simulink model "SIL_OlfatiSaber"  (R2021b)
settings: Solver=FixedStepDiscrete  StartTime=0  StopTime=T  FixedStep=0.01  RelTol=1e-3  EnableMultiTasking=on
model workspace (MAT data in the model file):
  SL_ROS_VariableLengthArrays_MaxSizes : object (value not decoded)
values from neighbouring files (symbols this model uses):
  airspeed_ref = 42    [start_swarm.m]
  altitude_ref = 300    [start_swarm.m]
  N_Waypoints = size(Waypoints,1)    [start_swarm.m]
  radius_waypoint = 200    [start_swarm.m]
  Waypoints = [1200 -1000 ... (first row only)    [start_swarm.m]
undefined symbols (not defined in the file or in its folder): DiscIntNeverNeededParam, Elevators, p_swarm, Propeller, RightAileron, RightFlap, Rudder
libraries: robotlib x36, slpidlib x15, eeGeneralControl x5, simulink x5
(part 2 of 5)

== system SIL_OlfatiSaber/UAV 2/High-level/Waypoint Generator ==
  Xi : Inport
  Pos_i : Inport  Port=2
  Constant : Constant  Value=radius_waypoint
  Constant1 : Constant  Value=Waypoints
  Constant2 : Constant  Value=N_Waypoints
  Constant3 : Constant  Value=p_swarm.r
  Display : Display
  Memory : Memory
  Velocity Direction : MATLAB Function  TreatAsAtomicUnit=on
  Waypoint Algorithm : MATLAB Function  TreatAsAtomicUnit=on
  u : Outport
  wires:
  Memory/1 -> Waypoint Algorithm/6("Current_Waypoint ")
  Constant1/1 -> Waypoint Algorithm/4(Waypoints)
  Xi/1 -> Waypoint Algorithm/1(Xi)
  Constant3/1 -> Waypoint Algorithm/3(p_swarm_r)
  Constant2/1 -> Waypoint Algorithm/5(N_Waypoints)
  Waypoint Algorithm/2(Current_Waypoint) -> Memory/1, Display/1
  Constant/1 -> Waypoint Algorithm/2(R)
  Pos_i/1 -> Velocity Direction/1(pos)
  Velocity Direction/1(u_ref) -> u/1
  Waypoint Algorithm/1(wp) -> Velocity Direction/2(wp)

== system SIL_OlfatiSaber/UAV 2/Low-level/Autopilot ==
  note: bota po
  vel ref : Inport
  Euler angles : Inport  Port=2
  roll_ref : Inport  Port=3
  altitude : Inport  Port=4
  vel_in : Inport  Port=5
  altitude ref : Inport  Port=6
  Altitude Control : Subsystem
      settings: PortSchema="{\"entries\":[{\"content\":{\"sides\":[{\"content\":{\"connectorIds\":[\"In1\",\"In2\"]},\"type\":\"ConnectorPlacement.EquallySpacedRectSide\",\"uuid\":\"98c80c82-2588-492a-897d-d133440579b3\"},{\"content\":{\"connectorIds\":[\"Out1\"],\"side\":\"RIGHT\"},\"type\":\"ConnectorPlacement.EquallySpacedRectSide\",\"uuid\":\"157fcffb-564d-4941-a636-42e4165df758\"},{\"content\":{\"connectorIds\":[\"Out2\"],\"side\":\"TOP\"},\"type\":\"ConnectorPlacement.EquallySpacedRectSide\",\"uuid\":\"44b57248-226e-45fd-814c-d7eb072c2d1f\"},{\"content\":{\"connectorIds\":[],\"side\":\"HIDDEN\"},\"type\":\"ConnectorPlacement.EquallySpacedRectSide\",\"uuid\":\"dff6d6ab-ae11-4516-9107-00b7ae45fb5b\"}]},\"type\":\"ConnectorPlacement.EquallySpacedConnector\",\"uuid\":\"b6a62117-e3d4-4c2a-a3b5-b134a2ba950a\"}],\"packageUris\":[\"http://schema.mathworks.com/mf0/Connector/R2020b\"],\"version\":\"1.0\"}"
  Attitude Control : Subsystem
  Constant : Constant  Value=0
  Saturation2 : Saturate  UpperLimit=0.0523599  LowerLimit=-0.0523599
  Saturation3 : Saturate  UpperLimit=0.8  LowerLimit=0.6
  Saturation4 : Saturate  UpperLimit=0.0523599  LowerLimit=-0.0523599
  Takeoff : Subsystem  Commented=on
  Velocity Control : Subsystem
      settings: PortSchema="{\"entries\":[{\"content\":{\"sides\":[{\"content\":{\"connectorIds\":[\"In1\",\"In2\"]},\"type\":\"ConnectorPlacement.EquallySpacedRectSide\",\"uuid\":\"98c80c82-2588-492a-897d-d133440579b3\"},{\"content\":{\"connectorIds\":[\"Out1\"],\"side\":\"RIGHT\"},\"type\":\"ConnectorPlacement.EquallySpacedRectSide\",\"uuid\":\"157fcffb-564d-4941-a636-42e4165df758\"},{\"content\":{\"connectorIds\":[\"Out2\"],\"side\":\"TOP\"},\"type\":\"ConnectorPlacement.EquallySpacedRectSide\",\"uuid\":\"44b57248-226e-45fd-814c-d7eb072c2d1f\"},{\"content\":{\"connectorIds\":[],\"side\":\"HIDDEN\"},\"type\":\"ConnectorPlacement.EquallySpacedRectSide\",\"uuid\":\"dff6d6ab-ae11-4516-9107-00b7ae45fb5b\"}]},\"type\":\"ConnectorPlacement.EquallySpacedConnector\",\"uuid\":\"b6a62117-e3d4-4c2a-a3b5-b134a2ba950a\"}],\"packageUris\":[\"http://schema.mathworks.com/mf0/Connector/R2020b\"],\"version\":\"1.0\"}"
  profundor_cmd : Outport
  rudder_cmd : Outport  Port=2
  aileron_cmd : Outport  Port=3
  propeller_cmd : Outport  Port=4
  alt_e : Outport  Port=5
  vel_e : Outport  Port=6
  roll_e : Outport  Port=7
  pitch_e : Outport  Port=8
  wires:
  vel ref/1 -> Velocity Control/1(Velocity Ref)
  altitude ref/1 -> Altitude Control/1(Altitude Ref)
  vel_in/1 -> Velocity Control/2(Velocity)
  Altitude Control/2(altitude_error) -> alt_e/1
  Velocity Control/2(velocity_error) -> vel_e/1
  Altitude Control/1(Pitch_ref) -> Attitude Control/1(Pitch Ref)
  roll_ref/1 -> Attitude Control/2(Roll_ref)
  Euler angles/1 -> Attitude Control/3(Euler angles)
  Attitude Control/1(pitch_error) -> pitch_e/1, Saturation4/1
  Attitude Control/2(roll_error) -> Saturation2/1, roll_e/1
  Velocity Control/1(propeller_cmd) -> Saturation3/1
  Saturation3/1 -> propeller_cmd/1
  Saturation2/1 -> aileron_cmd/1
  Saturation4/1 -> profundor_cmd/1
  altitude/1 -> Altitude Control/2(Altitude)
  Constant/1 -> rudder_cmd/1

== system SIL_OlfatiSaber/UAV 2/Low-level/Guidance Algorithm ==
  yaw : Inport
  x : Inport  Port=2
  y : Inport  Port=3
  x ref : Inport  Port=4
  y ref : Inport  Port=5
  Atan2 : Trigonometry  Operator=atan2
  Constant : Constant
  Constant1 : Constant  Value=0
  Constant2 : Constant  Value=1.2
  Constant3 : Constant  Value=10
  Discrete PID : slpidlib/PID Controller  Controller=PID  Form=Parallel  TimeDomain=Discrete-time  UseExternalTs=off  SampleTime=-1  IntegratorMethod=Forward Euler  FilterMethod=Forward Euler  ControllerParametersSource=external  P=1  I=1  D=0  UseFilter=on  N=100  TunerSelectOption=Transfer Function Based (PID Tuner App)  InitialConditionSource=internal  InitialConditionForIntegrator=0  InitialConditionForFilter=0  DifferentiatorICPrevScaledInput=0  ExternalReset=none  TrackingMode=off  Kt=1  LimitOutput=off  SatLimitsSource=internal  UpperSaturationLimit=inf  LowerSaturationLimit=-inf  LinearizeAsGain=on  AntiWindupMode=none  Kb=1  POutMin=[]  POutMax=[]  IOutMin=[]  IOutMax=[]  DOutMin=[]  DOutMax=[]  NOutMin=[]  NOutMax=[]  SumOutMin=[]  SumOutMax=[]  SaturationOutMin=[]  SaturationOutMax=[]  PParamMin=[]  PParamMax=[]  IParamMin=[]  IParamMax=[]  DParamMin=[]  DParamMax=[]  NParamMin=[]  NParamMax=[]  KbParamMin=[]  KbParamMax=[]  KtParamMin=[]  KtParamMax=[]  KbOutMin=[]  KbOutMax=[]  KtOutMin=[]  KtOutMax=[]  IntegratorOutMin=[]  IntegratorOutMax=[]  FilterOutMin=[]  FilterOutMax=[]  SumI1OutMin=[]  SumI1OutMax=[]  SumI2OutMin=[]  SumI2OutMax=[]  SumI3OutMin=[]  SumI3OutMax=[]  SumI4OutMin=[]  SumI4OutMax=[]  SumDOutMin=[]  SumDOutMax=[]  DifferentiatorOutMin=[]  DifferentiatorOutMax=[]  FilterDiffOutCoefMin=[]  FilterDiffOutCoefMax=[]  ReciprocalOutMin=[]  ReciprocalOutMax=[]  SumDenOutMin=[]  SumDenOutMax=[]  SumNumOutMin=[]  SumNumOutMax=[]  DivideOutMin=[]  DivideOutMax=[]  UdiffTsProdOutMin=[]  UdiffTsProdOutMax=[]  NTsProdOutMin=[]  NTsProdOutMax=[]  UintegralTsProdOutMin=[]  UintegralTsProdOutMax=[]  UngainTsProdOutMin=[]  UngainTsProdOutMax=[]  IntegratorContinuousStateAttributes=''  IntegratorStateMustResolveToSignalObject=off  IntegratorRTWStateStorageClass=Auto  FilterContinuousStateAttributes=''  FilterStateMustResolveToSignalObject=off  FilterRTWStateStorageClass=Auto  ParallelPVariant=ExternalParameters  IdealPVariant=Disabled  IVariant=ExternalParameters  DVariant=ExternalParameters  IntegratorVariant=Discrete  SatVariant=Disabled  AWVariant=Passthrough  PCopyVariant=Disabled  TRVariant=Disabled  FdbkBlocksVariant=Forward  IdealPFdbkVariant=Disabled  SatFdbkVariant=Disabled  DerivativeFilterVariant=ForwardEulerFilter  NVariant=ExternalParameters  NCopyVariant=Disabled  FilterICVariant=InternalICsFilter  IntegratorICVariant=InternalICs  ExternalResetVariant=Disabled  TRSumVariant=Passthrough  SumFdbkVariant=Disabled  SumVariant=Sum_PID  TsampFilterVariant=InternalTs  TsampNgainVariant=Passthrough  TsampIntegralVariant=Passthrough  ExternalSaturationOutDataTypeStr=Inherit: Same as second input
  Gain : Gain  Gain=1.67
  Gain1 : Gain  Gain=-1
  Mux1 : Mux  Inputs=2
  Mux2 : Mux  Inputs=2
  Mux3 : Mux  Inputs=2
  Saturation : Saturate  UpperLimit=0.226893  LowerLimit=-0.226893
  Sum2 : Sum  Inputs=|+-
  Sum3 : Sum  Inputs=|+-
  Sum4 : Sum  Inputs=|+-
  roll_ref : Outport
  yaw_error : Outport  Port=2
  positions : Outport  Port=3
  wires:
  Mux1/1 -> Mux3/1
  Mux2/1 -> Mux3/2
  Saturation/1 -> Gain1/1
  Sum3/1 -> Atan2/1
  y/1 -> Sum3/2, Mux2/2
  y ref/1 -> Mux2/1, Sum3/1
  x ref/1 -> Mux1/1, Sum2/1
  x/1 -> Sum2/2, Mux1/2
  Sum2/1 -> Atan2/2
  Atan2/1 -> Sum4/1
  yaw/1 -> Sum4/2
  Mux3/1 -> positions/1
  Discrete PID/1 -> Saturation/1
  Sum4/1 -> yaw_error/1, Gain/1
  Gain1/1 -> roll_ref/1
  Constant/1 -> Discrete PID/2
  Constant1/1 -> Discrete PID/3
  Constant2/1 -> Discrete PID/4
  Constant3/1 -> Discrete PID/5
  Gain/1 -> Discrete PID/1

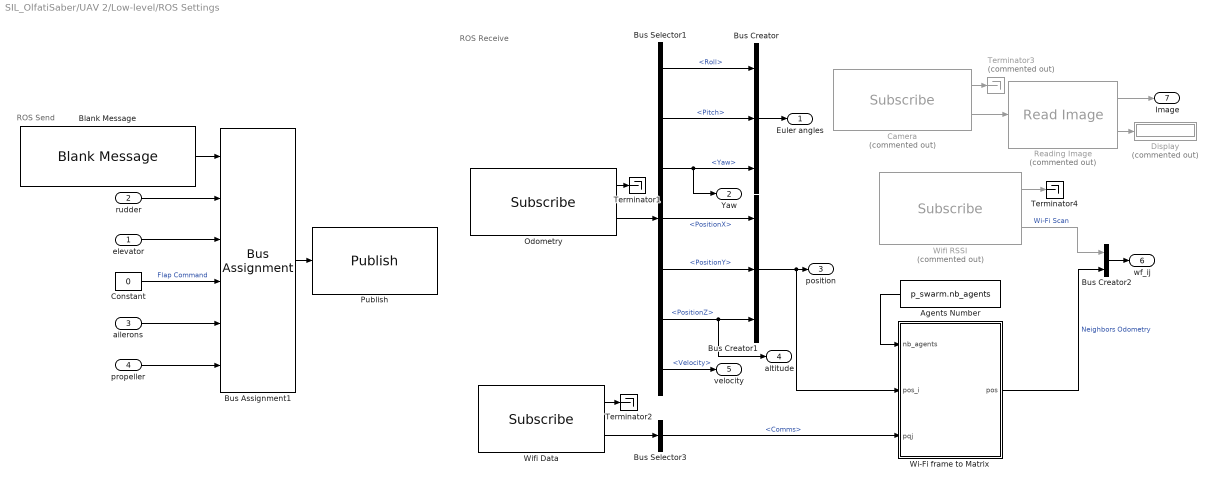
== system SIL_OlfatiSaber/UAV 2/Low-level/ROS Settings ==
  note: ROS Receive
  note: ROS Send
  elevator : Inport
  rudder : Inport  Port=2
  ailerons : Inport  Port=3
  propeller : Inport  Port=4
  Agents Number : Constant  Value=p_swarm.nb_agents
  Blank Message : robotlib/Blank Message  messageClass=Message  entityType=cosmus_messages/Control_Surfaces  messageType=cosmus_messages/Control_Surfaces  SampleTime=-1  legacyBusStruct=off
  Bus Assignment1 : BusAssignment  AssignedSignals=Rudder,Elevators,RightFlap,RightAileron,Propeller
  Bus Creator : BusCreator  Inputs=3
  Bus Creator1 : BusCreator  Inputs=3
  Bus Creator2 : BusCreator  Inputs=2
  Bus Selector1 : BusSelector  OutputSignals=Roll,Pitch,Yaw,PositionX,PositionY,PositionZ,Velocity
  Bus Selector3 : BusSelector  OutputSignals=Comms
  Camera : robotlib/Subscribe  Commented=on  topicSource=Select from ROS network  topic=/uav1/camera/image_raw  messageType=sensor_msgs/Image  SampleTime=-1  legacyBusStruct=off  messageQueueLength=1
  Constant : Constant  Value=0
  Display : Display  Commented=on
  Odometry : robotlib/Subscribe  topicSource=Select from ROS network  topic=/uav2/ground_truth/Odometry  messageType=cosmus_communication/Odom  SampleTime=-1  legacyBusStruct=off  messageQueueLength=1
  Publish : robotlib/Publish  topicSource=Select from ROS network  topic=/uav2/command  messageType=cosmus_messages/Control_Surfaces  legacyBusStruct=off  messageQueueLength=1
  Reading Image : robotlib/Read Image  Commented=on  MaximumImageSize=[240, 360]  ImageEncoding=rgb8  ShowAlphaOutput=off  ShowErrorCodeOutput=on  VariableSizeOutputs=off
      settings: SourceProductBaseCode=RR
  Terminator1 : Terminator
  Terminator2 : Terminator
  Terminator3 : Terminator  Commented=on
  Terminator4 : Terminator
  Wi-Fi frame to Matrix : MATLAB Function  TreatAsAtomicUnit=on
  Wifi Data : robotlib/Subscribe  topicSource=Select from ROS network  topic=/uav2/wifi_receiver/data  messageType=cosmus_messages/NetworkComm  SampleTime=-1  legacyBusStruct=off  messageQueueLength=1
  Wifi RSSI : robotlib/Subscribe  Commented=on  topicSource=Select from ROS network  topic=/uav1/wifi_receiver/wifi_scan  messageType=cosmus_messages/WifiSignals  SampleTime=-1  legacyBusStruct=off  messageQueueLength=1
  Euler angles : Outport
  Yaw : Outport  Port=2
  position : Outport  Port=3
  altitude : Outport  Port=4
  velocity : Outport  Port=5
  wf_ij : Outport  Port=6
  Image : Outport  Port=7
  wires:
  Odometry/1 -> Terminator1/1
  Blank Message/1 -> Bus Assignment1/1
  Bus Selector1/3 -> Bus Creator/3, Yaw/1  "<Yaw>"
  Bus Creator/1 -> Euler angles/1
  Bus Selector1/1 -> Bus Creator/1  "<Roll>"
  Bus Selector1/2 -> Bus Creator/2  "<Pitch>"
  Constant/1 -> Bus Assignment1/4  "Flap Command"
  Bus Assignment1/1 -> Publish/1
  Odometry/2 -> Bus Selector1/1
  Bus Selector1/4 -> Bus Creator1/1  "<PositionX>"
  Bus Selector1/5 -> Bus Creator1/2  "<PositionY>"
  Bus Selector1/6 -> Bus Creator1/3, altitude/1  "<PositionZ>"
  propeller/1 -> Bus Assignment1/6
  ailerons/1 -> Bus Assignment1/5
  elevator/1 -> Bus Assignment1/3
  Bus Selector1/7 -> velocity/1  "<Velocity>"
  rudder/1 -> Bus Assignment1/2
  Wifi Data/1 -> Terminator2/1
  Wifi Data/2 -> Bus Selector3/1
  Bus Selector3/1 -> Wi-Fi frame to Matrix/3(pqj)  "<Comms>"
  Agents Number/1 -> Wi-Fi frame to Matrix/1(nb_agents)
  Bus Creator1/1 -> position/1, Wi-Fi frame to Matrix/2(pos_i)
  Wi-Fi frame to Matrix/1(pos) -> Bus Creator2/2  "Neighbors Odometry"
  Camera/2 -> Reading Image/1
  Reading Image/1 -> Image/1
  Reading Image/2 -> Display/1
  Camera/1 -> Terminator3/1
  Wifi RSSI/1 -> Terminator4/1
  Wifi RSSI/2 -> Bus Creator2/1  "Wi-Fi Scan"
  Bus Creator2/1 -> wf_ij/1

== system SIL_OlfatiSaber/UAV 2/Low-level/Vision ==
  Image : Inport
  Video Viewer : VideoViewer  Commented=on  FigPos=[505 744 418 304]
  wires:
  Image/1 -> Video Viewer/1

== system SIL_OlfatiSaber/UAV 3/High-level/Coordination Algorithm ==
  Xi : Inport
  u : Inport  Port=2
  Demux : Demux  Outputs=3
  Discrete Derivative : simulink/Discrete/Discrete Derivative  gainval=1.0  ICPrevScaledInput=0.0  OutMin=[]  OutMax=[]  OutDataType=fixdt(1, 16)  OutScaling=2^-10  DoSatur=off
  Discrete-Time Integrator : DiscreteIntegrator  SampleTime=-1  ICPrevOutput=DiscIntNeverNeededParam  ICPrevScaledInput=DiscIntNeverNeededParam
  Olfati-Saber Algorithm : MATLAB Function  TreatAsAtomicUnit=on
  Parameters : Subsystem
  dt : Constant  Value=0.01
  r_agent : Constant  Value=p_swarm.r_agent
  X : Outport
  Y : Outport  Port=2
  Z : Outport  Port=3
  wires:
  Olfati-Saber Algorithm/1(vel_command) -> Discrete-Time Integrator/1
  dt/1 -> Olfati-Saber Algorithm/5(dt)
  r_agent/1 -> Olfati-Saber Algorithm/6(r_agent)
  Discrete-Time Integrator/1 -> Demux/1
  Demux/2 -> Y/1
  Demux/1 -> X/1
  Demux/3 -> Z/1
  Discrete Derivative/1 -> Olfati-Saber Algorithm/3(vel)
  Parameters/1(p_swarm) -> Olfati-Saber Algorithm/1(p_swarm_par)
  Xi/1 -> Discrete Derivative/1, Olfati-Saber Algorithm/2(pos)
  u/1 -> Olfati-Saber Algorithm/4(u_ref)

== system SIL_OlfatiSaber/UAV 3/High-level/Network ==
  Scan : Inport
  Agents Number : Constant  Value=p_swarm.nb_agents
  Bus Selector : BusSelector  OutputSignals=Neighbors Odometry,Wi-Fi Scan
  Status Network : MATLAB Function  Commented=on  TreatAsAtomicUnit=on
  Terminator5 : Terminator
  Pos_J : Outport
  wires:
  Status Network/1(SignalDbms) -> Terminator5/1
  Agents Number/1 -> Status Network/1(N_Agents)
  Scan/1 -> Bus Selector/1
  Bus Selector/1 -> Pos_J/1  "<Neighbors Odometry>"
  Bus Selector/2 -> Status Network/2(Wifi_Scan)  "<Wi-Fi Scan>"

== system SIL_OlfatiSaber/UAV 3/High-level/Waypoint Generator ==
  Xi : Inport
  Pos_i : Inport  Port=2
  Constant : Constant  Value=radius_waypoint
  Constant1 : Constant  Value=Waypoints
  Constant2 : Constant  Value=N_Waypoints
  Constant3 : Constant  Value=p_swarm.r
  Display : Display
  Memory : Memory
  Velocity Direction : MATLAB Function  TreatAsAtomicUnit=on
  Waypoint Algorithm : MATLAB Function  TreatAsAtomicUnit=on
  u : Outport
  wires:
  Memory/1 -> Waypoint Algorithm/6("Current_Waypoint ")
  Constant1/1 -> Waypoint Algorithm/4(Waypoints)
  Xi/1 -> Waypoint Algorithm/1(Xi)
  Constant3/1 -> Waypoint Algorithm/3(p_swarm_r)
  Constant2/1 -> Waypoint Algorithm/5(N_Waypoints)
  Waypoint Algorithm/2(Current_Waypoint) -> Memory/1, Display/1
  Constant/1 -> Waypoint Algorithm/2(R)
  Pos_i/1 -> Velocity Direction/1(pos)
  Velocity Direction/1(u_ref) -> u/1
  Waypoint Algorithm/1(wp) -> Velocity Direction/2(wp)

== system SIL_OlfatiSaber/UAV 3/Low-level/Autopilot ==
  note: bota po
  vel ref : Inport
  Euler angles : Inport  Port=2
  roll_ref : Inport  Port=3
  altitude : Inport  Port=4
  vel_in : Inport  Port=5
  altitude ref : Inport  Port=6
  Altitude Control : Subsystem
      settings: PortSchema="{\"entries\":[{\"content\":{\"sides\":[{\"content\":{\"connectorIds\":[\"In1\",\"In2\"]},\"type\":\"ConnectorPlacement.EquallySpacedRectSide\",\"uuid\":\"98c80c82-2588-492a-897d-d133440579b3\"},{\"content\":{\"connectorIds\":[\"Out1\"],\"side\":\"RIGHT\"},\"type\":\"ConnectorPlacement.EquallySpacedRectSide\",\"uuid\":\"157fcffb-564d-4941-a636-42e4165df758\"},{\"content\":{\"connectorIds\":[\"Out2\"],\"side\":\"TOP\"},\"type\":\"ConnectorPlacement.EquallySpacedRectSide\",\"uuid\":\"44b57248-226e-45fd-814c-d7eb072c2d1f\"},{\"content\":{\"connectorIds\":[],\"side\":\"HIDDEN\"},\"type\":\"ConnectorPlacement.EquallySpacedRectSide\",\"uuid\":\"dff6d6ab-ae11-4516-9107-00b7ae45fb5b\"}]},\"type\":\"ConnectorPlacement.EquallySpacedConnector\",\"uuid\":\"b6a62117-e3d4-4c2a-a3b5-b134a2ba950a\"}],\"packageUris\":[\"http://schema.mathworks.com/mf0/Connector/R2020b\"],\"version\":\"1.0\"}"
  Attitude Control : Subsystem
  Constant : Constant  Value=0
  Saturation2 : Saturate  UpperLimit=0.0523599  LowerLimit=-0.0523599
  Saturation3 : Saturate  UpperLimit=0.8  LowerLimit=0.6
  Saturation4 : Saturate  UpperLimit=0.0523599  LowerLimit=-0.0523599
  Takeoff : Subsystem  Commented=on
  Velocity Control : Subsystem
      settings: PortSchema="{\"entries\":[{\"content\":{\"sides\":[{\"content\":{\"connectorIds\":[\"In1\",\"In2\"]},\"type\":\"ConnectorPlacement.EquallySpacedRectSide\",\"uuid\":\"98c80c82-2588-492a-897d-d133440579b3\"},{\"content\":{\"connectorIds\":[\"Out1\"],\"side\":\"RIGHT\"},\"type\":\"ConnectorPlacement.EquallySpacedRectSide\",\"uuid\":\"157fcffb-564d-4941-a636-42e4165df758\"},{\"content\":{\"connectorIds\":[\"Out2\"],\"side\":\"TOP\"},\"type\":\"ConnectorPlacement.EquallySpacedRectSide\",\"uuid\":\"44b57248-226e-45fd-814c-d7eb072c2d1f\"},{\"content\":{\"connectorIds\":[],\"side\":\"HIDDEN\"},\"type\":\"ConnectorPlacement.EquallySpacedRectSide\",\"uuid\":\"dff6d6ab-ae11-4516-9107-00b7ae45fb5b\"}]},\"type\":\"ConnectorPlacement.EquallySpacedConnector\",\"uuid\":\"b6a62117-e3d4-4c2a-a3b5-b134a2ba950a\"}],\"packageUris\":[\"http://schema.mathworks.com/mf0/Connector/R2020b\"],\"version\":\"1.0\"}"
  profundor_cmd : Outport
  rudder_cmd : Outport  Port=2
  aileron_cmd : Outport  Port=3
  propeller_cmd : Outport  Port=4
  alt_e : Outport  Port=5
  vel_e : Outport  Port=6
  roll_e : Outport  Port=7
  pitch_e : Outport  Port=8
  wires:
  vel ref/1 -> Velocity Control/1(Velocity Ref)
  altitude ref/1 -> Altitude Control/1(Altitude Ref)
  vel_in/1 -> Velocity Control/2(Velocity)
  Altitude Control/2(altitude_error) -> alt_e/1
  Velocity Control/2(velocity_error) -> vel_e/1
  Altitude Control/1(Pitch_ref) -> Attitude Control/1(Pitch Ref)
  roll_ref/1 -> Attitude Control/2(Roll_ref)
  Euler angles/1 -> Attitude Control/3(Euler angles)
  Attitude Control/1(pitch_error) -> pitch_e/1, Saturation4/1
  Attitude Control/2(roll_error) -> Saturation2/1, roll_e/1
  Velocity Control/1(propeller_cmd) -> Saturation3/1
  Saturation3/1 -> propeller_cmd/1
  Saturation2/1 -> aileron_cmd/1
  Saturation4/1 -> profundor_cmd/1
  altitude/1 -> Altitude Control/2(Altitude)
  Constant/1 -> rudder_cmd/1

== system SIL_OlfatiSaber/UAV 3/Low-level/Guidance Algorithm ==
  yaw : Inport
  x : Inport  Port=2
  y : Inport  Port=3
  x ref : Inport  Port=4
  y ref : Inport  Port=5
  Atan2 : Trigonometry  Operator=atan2
  Constant : Constant
  Constant1 : Constant  Value=0
  Constant2 : Constant  Value=1.2
  Constant3 : Constant  Value=10
  Discrete PID : slpidlib/PID Controller  Controller=PID  Form=Parallel  TimeDomain=Discrete-time  UseExternalTs=off  SampleTime=-1  IntegratorMethod=Forward Euler  FilterMethod=Forward Euler  ControllerParametersSource=external  P=1  I=1  D=0  UseFilter=on  N=100  TunerSelectOption=Transfer Function Based (PID Tuner App)  InitialConditionSource=internal  InitialConditionForIntegrator=0  InitialConditionForFilter=0  DifferentiatorICPrevScaledInput=0  ExternalReset=none  TrackingMode=off  Kt=1  LimitOutput=off  SatLimitsSource=internal  UpperSaturationLimit=inf  LowerSaturationLimit=-inf  LinearizeAsGain=on  AntiWindupMode=none  Kb=1  POutMin=[]  POutMax=[]  IOutMin=[]  IOutMax=[]  DOutMin=[]  DOutMax=[]  NOutMin=[]  NOutMax=[]  SumOutMin=[]  SumOutMax=[]  SaturationOutMin=[]  SaturationOutMax=[]  PParamMin=[]  PParamMax=[]  IParamMin=[]  IParamMax=[]  DParamMin=[]  DParamMax=[]  NParamMin=[]  NParamMax=[]  KbParamMin=[]  KbParamMax=[]  KtParamMin=[]  KtParamMax=[]  KbOutMin=[]  KbOutMax=[]  KtOutMin=[]  KtOutMax=[]  IntegratorOutMin=[]  IntegratorOutMax=[]  FilterOutMin=[]  FilterOutMax=[]  SumI1OutMin=[]  SumI1OutMax=[]  SumI2OutMin=[]  SumI2OutMax=[]  SumI3OutMin=[]  SumI3OutMax=[]  SumI4OutMin=[]  SumI4OutMax=[]  SumDOutMin=[]  SumDOutMax=[]  DifferentiatorOutMin=[]  DifferentiatorOutMax=[]  FilterDiffOutCoefMin=[]  FilterDiffOutCoefMax=[]  ReciprocalOutMin=[]  ReciprocalOutMax=[]  SumDenOutMin=[]  SumDenOutMax=[]  SumNumOutMin=[]  SumNumOutMax=[]  DivideOutMin=[]  DivideOutMax=[]  UdiffTsProdOutMin=[]  UdiffTsProdOutMax=[]  NTsProdOutMin=[]  NTsProdOutMax=[]  UintegralTsProdOutMin=[]  UintegralTsProdOutMax=[]  UngainTsProdOutMin=[]  UngainTsProdOutMax=[]  IntegratorContinuousStateAttributes=''  IntegratorStateMustResolveToSignalObject=off  IntegratorRTWStateStorageClass=Auto  FilterContinuousStateAttributes=''  FilterStateMustResolveToSignalObject=off  FilterRTWStateStorageClass=Auto  ParallelPVariant=ExternalParameters  IdealPVariant=Disabled  IVariant=ExternalParameters  DVariant=ExternalParameters  IntegratorVariant=Discrete  SatVariant=Disabled  AWVariant=Passthrough  PCopyVariant=Disabled  TRVariant=Disabled  FdbkBlocksVariant=Forward  IdealPFdbkVariant=Disabled  SatFdbkVariant=Disabled  DerivativeFilterVariant=ForwardEulerFilter  NVariant=ExternalParameters  NCopyVariant=Disabled  FilterICVariant=InternalICsFilter  IntegratorICVariant=InternalICs  ExternalResetVariant=Disabled  TRSumVariant=Passthrough  SumFdbkVariant=Disabled  SumVariant=Sum_PID  TsampFilterVariant=InternalTs  TsampNgainVariant=Passthrough  TsampIntegralVariant=Passthrough  ExternalSaturationOutDataTypeStr=Inherit: Same as second input
  Gain : Gain  Gain=1.67
  Gain1 : Gain  Gain=-1
  Mux1 : Mux  Inputs=2
  Mux2 : Mux  Inputs=2
  Mux3 : Mux  Inputs=2
  Saturation : Saturate  UpperLimit=0.226893  LowerLimit=-0.226893
  Sum2 : Sum  Inputs=|+-
  Sum3 : Sum  Inputs=|+-
  Sum4 : Sum  Inputs=|+-
  roll_ref : Outport
  yaw_error : Outport  Port=2
  positions : Outport  Port=3
  wires:
  Mux1/1 -> Mux3/1
  Mux2/1 -> Mux3/2
  Saturation/1 -> Gain1/1
  Sum3/1 -> Atan2/1
  y/1 -> Sum3/2, Mux2/2
  y ref/1 -> Mux2/1, Sum3/1
  x ref/1 -> Mux1/1, Sum2/1
  x/1 -> Sum2/2, Mux1/2
  Sum2/1 -> Atan2/2
  Atan2/1 -> Sum4/1
  yaw/1 -> Sum4/2
  Mux3/1 -> positions/1
  Discrete PID/1 -> Saturation/1
  Sum4/1 -> yaw_error/1, Gain/1
  Gain1/1 -> roll_ref/1
  Constant/1 -> Discrete PID/2
  Constant1/1 -> Discrete PID/3
  Constant2/1 -> Discrete PID/4
  Constant3/1 -> Discrete PID/5
  Gain/1 -> Discrete PID/1

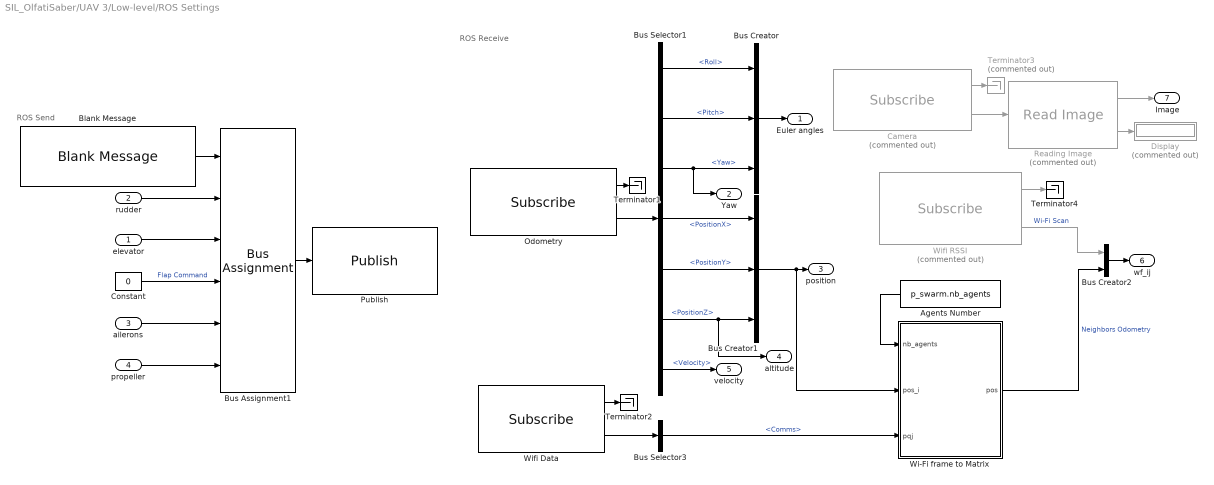
== system SIL_OlfatiSaber/UAV 3/Low-level/ROS Settings ==
  note: ROS Receive
  note: ROS Send
  elevator : Inport
  rudder : Inport  Port=2
  ailerons : Inport  Port=3
  propeller : Inport  Port=4
  Agents Number : Constant  Value=p_swarm.nb_agents
  Blank Message : robotlib/Blank Message  messageClass=Message  entityType=cosmus_messages/Control_Surfaces  messageType=cosmus_messages/Control_Surfaces  SampleTime=-1  legacyBusStruct=off
  Bus Assignment1 : BusAssignment  AssignedSignals=Rudder,Elevators,RightFlap,RightAileron,Propeller
  Bus Creator : BusCreator  Inputs=3
  Bus Creator1 : BusCreator  Inputs=3
  Bus Creator2 : BusCreator  Inputs=2
  Bus Selector1 : BusSelector  OutputSignals=Roll,Pitch,Yaw,PositionX,PositionY,PositionZ,Velocity
  Bus Selector3 : BusSelector  OutputSignals=Comms
  Camera : robotlib/Subscribe  Commented=on  topicSource=Select from ROS network  topic=/uav1/camera/image_raw  messageType=sensor_msgs/Image  SampleTime=-1  legacyBusStruct=off  messageQueueLength=1
  Constant : Constant  Value=0
  Display : Display  Commented=on
  Odometry : robotlib/Subscribe  topicSource=Select from ROS network  topic=/uav3/ground_truth/Odometry  messageType=cosmus_communication/Odom  SampleTime=-1  legacyBusStruct=off  messageQueueLength=1
  Publish : robotlib/Publish  topicSource=Select from ROS network  topic=/uav3/command  messageType=cosmus_messages/Control_Surfaces  legacyBusStruct=off  messageQueueLength=1
  Reading Image : robotlib/Read Image  Commented=on  MaximumImageSize=[240, 360]  ImageEncoding=rgb8  ShowAlphaOutput=off  ShowErrorCodeOutput=on  VariableSizeOutputs=off
      settings: SourceProductBaseCode=RR
  Terminator1 : Terminator
  Terminator2 : Terminator
  Terminator3 : Terminator  Commented=on
  Terminator4 : Terminator
  Wi-Fi frame to Matrix : MATLAB Function  TreatAsAtomicUnit=on
  Wifi Data : robotlib/Subscribe  topicSource=Select from ROS network  topic=/uav3/wifi_receiver/data  messageType=cosmus_messages/NetworkComm  SampleTime=-1  legacyBusStruct=off  messageQueueLength=1
  Wifi RSSI : robotlib/Subscribe  Commented=on  topicSource=Select from ROS network  topic=/uav1/wifi_receiver/wifi_scan  messageType=cosmus_messages/WifiSignals  SampleTime=-1  legacyBusStruct=off  messageQueueLength=1
  Euler angles : Outport
  Yaw : Outport  Port=2
  position : Outport  Port=3
  altitude : Outport  Port=4
  velocity : Outport  Port=5
  wf_ij : Outport  Port=6
  Image : Outport  Port=7
  wires:
  Odometry/1 -> Terminator1/1
  Blank Message/1 -> Bus Assignment1/1
  Bus Selector1/3 -> Bus Creator/3, Yaw/1  "<Yaw>"
  Bus Creator/1 -> Euler angles/1
  Bus Selector1/1 -> Bus Creator/1  "<Roll>"
  Bus Selector1/2 -> Bus Creator/2  "<Pitch>"
  Constant/1 -> Bus Assignment1/4  "Flap Command"
  Bus Assignment1/1 -> Publish/1
  Odometry/2 -> Bus Selector1/1
  Bus Selector1/4 -> Bus Creator1/1  "<PositionX>"
  Bus Selector1/5 -> Bus Creator1/2  "<PositionY>"
  Bus Selector1/6 -> Bus Creator1/3, altitude/1  "<PositionZ>"
  propeller/1 -> Bus Assignment1/6
  ailerons/1 -> Bus Assignment1/5
  elevator/1 -> Bus Assignment1/3
  Bus Selector1/7 -> velocity/1  "<Velocity>"
  rudder/1 -> Bus Assignment1/2
  Wifi Data/1 -> Terminator2/1
  Wifi Data/2 -> Bus Selector3/1
  Bus Selector3/1 -> Wi-Fi frame to Matrix/3(pqj)  "<Comms>"
  Agents Number/1 -> Wi-Fi frame to Matrix/1(nb_agents)
  Bus Creator1/1 -> position/1, Wi-Fi frame to Matrix/2(pos_i)
  Wi-Fi frame to Matrix/1(pos) -> Bus Creator2/2  "Neighbors Odometry"
  Camera/2 -> Reading Image/1
  Reading Image/1 -> Image/1
  Reading Image/2 -> Display/1
  Camera/1 -> Terminator3/1
  Wifi RSSI/1 -> Terminator4/1
  Wifi RSSI/2 -> Bus Creator2/1  "Wi-Fi Scan"
  Bus Creator2/1 -> wf_ij/1

== system SIL_OlfatiSaber/UAV 3/Low-level/Vision ==
  Image : Inport
  Video Viewer : VideoViewer  Commented=on  FigPos=[505 744 418 304]
  wires:
  Image/1 -> Video Viewer/1

== system SIL_OlfatiSaber/UAV 4/High-level/Coordination Algorithm ==
  Xi : Inport
  u : Inport  Port=2
  Demux : Demux  Outputs=3
  Discrete Derivative : simulink/Discrete/Discrete Derivative  gainval=1.0  ICPrevScaledInput=0.0  OutMin=[]  OutMax=[]  OutDataType=fixdt(1, 16)  OutScaling=2^-10  DoSatur=off
  Discrete-Time Integrator : DiscreteIntegrator  SampleTime=-1  ICPrevOutput=DiscIntNeverNeededParam  ICPrevScaledInput=DiscIntNeverNeededParam
  Olfati-Saber Algorithm : MATLAB Function  TreatAsAtomicUnit=on
  Parameters : Subsystem
  dt : Constant  Value=0.01
  r_agent : Constant  Value=p_swarm.r_agent
  X : Outport
  Y : Outport  Port=2
  Z : Outport  Port=3
  wires:
  Olfati-Saber Algorithm/1(vel_command) -> Discrete-Time Integrator/1
  dt/1 -> Olfati-Saber Algorithm/5(dt)
  r_agent/1 -> Olfati-Saber Algorithm/6(r_agent)
  Discrete-Time Integrator/1 -> Demux/1
  Demux/2 -> Y/1
  Demux/1 -> X/1
  Demux/3 -> Z/1
  Discrete Derivative/1 -> Olfati-Saber Algorithm/3(vel)
  Parameters/1(p_swarm) -> Olfati-Saber Algorithm/1(p_swarm_par)
  Xi/1 -> Discrete Derivative/1, Olfati-Saber Algorithm/2(pos)
  u/1 -> Olfati-Saber Algorithm/4(u_ref)

== system SIL_OlfatiSaber/UAV 4/High-level/Network ==
  Scan : Inport
  Agents Number : Constant  Value=p_swarm.nb_agents
  Bus Selector : BusSelector  OutputSignals=Neighbors Odometry,Wi-Fi Scan
  Status Network : MATLAB Function  Commented=on  TreatAsAtomicUnit=on
  Terminator5 : Terminator
  Pos_J : Outport
  wires:
  Status Network/1(SignalDbms) -> Terminator5/1
  Agents Number/1 -> Status Network/1(N_Agents)
  Scan/1 -> Bus Selector/1
  Bus Selector/1 -> Pos_J/1  "<Neighbors Odometry>"
  Bus Selector/2 -> Status Network/2(Wifi_Scan)  "<Wi-Fi Scan>"

== system SIL_OlfatiSaber/UAV 4/High-level/Waypoint Generator ==
  Xi : Inport
  Pos_i : Inport  Port=2
  Constant : Constant  Value=radius_waypoint
  Constant1 : Constant  Value=Waypoints
  Constant2 : Constant  Value=N_Waypoints
  Constant3 : Constant  Value=p_swarm.r
  Display : Display
  Memory : Memory
  Velocity Direction : MATLAB Function  TreatAsAtomicUnit=on
  Waypoint Algorithm : MATLAB Function  TreatAsAtomicUnit=on
  u : Outport
  wires:
  Memory/1 -> Waypoint Algorithm/6("Current_Waypoint ")
  Constant1/1 -> Waypoint Algorithm/4(Waypoints)
  Xi/1 -> Waypoint Algorithm/1(Xi)
  Constant3/1 -> Waypoint Algorithm/3(p_swarm_r)
  Constant2/1 -> Waypoint Algorithm/5(N_Waypoints)
  Waypoint Algorithm/2(Current_Waypoint) -> Memory/1, Display/1
  Constant/1 -> Waypoint Algorithm/2(R)
  Pos_i/1 -> Velocity Direction/1(pos)
  Velocity Direction/1(u_ref) -> u/1
  Waypoint Algorithm/1(wp) -> Velocity Direction/2(wp)

== system SIL_OlfatiSaber/UAV 4/Low-level/Autopilot ==
  note: bota po
  vel ref : Inport
  Euler angles : Inport  Port=2
  roll_ref : Inport  Port=3
  altitude : Inport  Port=4
  vel_in : Inport  Port=5
  altitude ref : Inport  Port=6
  Altitude Control : Subsystem
      settings: PortSchema="{\"entries\":[{\"content\":{\"sides\":[{\"content\":{\"connectorIds\":[\"In1\",\"In2\"]},\"type\":\"ConnectorPlacement.EquallySpacedRectSide\",\"uuid\":\"98c80c82-2588-492a-897d-d133440579b3\"},{\"content\":{\"connectorIds\":[\"Out1\"],\"side\":\"RIGHT\"},\"type\":\"ConnectorPlacement.EquallySpacedRectSide\",\"uuid\":\"157fcffb-564d-4941-a636-42e4165df758\"},{\"content\":{\"connectorIds\":[\"Out2\"],\"side\":\"TOP\"},\"type\":\"ConnectorPlacement.EquallySpacedRectSide\",\"uuid\":\"44b57248-226e-45fd-814c-d7eb072c2d1f\"},{\"content\":{\"connectorIds\":[],\"side\":\"HIDDEN\"},\"type\":\"ConnectorPlacement.EquallySpacedRectSide\",\"uuid\":\"dff6d6ab-ae11-4516-9107-00b7ae45fb5b\"}]},\"type\":\"ConnectorPlacement.EquallySpacedConnector\",\"uuid\":\"b6a62117-e3d4-4c2a-a3b5-b134a2ba950a\"}],\"packageUris\":[\"http://schema.mathworks.com/mf0/Connector/R2020b\"],\"version\":\"1.0\"}"
  Attitude Control : Subsystem
  Constant : Constant  Value=0
  Saturation2 : Saturate  UpperLimit=0.0523599  LowerLimit=-0.0523599
  Saturation3 : Saturate  UpperLimit=0.8  LowerLimit=0.6
  Saturation4 : Saturate  UpperLimit=0.0523599  LowerLimit=-0.0523599
  Takeoff : Subsystem  Commented=on
  Velocity Control : Subsystem
      settings: PortSchema="{\"entries\":[{\"content\":{\"sides\":[{\"content\":{\"connectorIds\":[\"In1\",\"In2\"]},\"type\":\"ConnectorPlacement.EquallySpacedRectSide\",\"uuid\":\"98c80c82-2588-492a-897d-d133440579b3\"},{\"content\":{\"connectorIds\":[\"Out1\"],\"side\":\"RIGHT\"},\"type\":\"ConnectorPlacement.EquallySpacedRectSide\",\"uuid\":\"157fcffb-564d-4941-a636-42e4165df758\"},{\"content\":{\"connectorIds\":[\"Out2\"],\"side\":\"TOP\"},\"type\":\"ConnectorPlacement.EquallySpacedRectSide\",\"uuid\":\"44b57248-226e-45fd-814c-d7eb072c2d1f\"},{\"content\":{\"connectorIds\":[],\"side\":\"HIDDEN\"},\"type\":\"ConnectorPlacement.EquallySpacedRectSide\",\"uuid\":\"dff6d6ab-ae11-4516-9107-00b7ae45fb5b\"}]},\"type\":\"ConnectorPlacement.EquallySpacedConnector\",\"uuid\":\"b6a62117-e3d4-4c2a-a3b5-b134a2ba950a\"}],\"packageUris\":[\"http://schema.mathworks.com/mf0/Connector/R2020b\"],\"version\":\"1.0\"}"
  profundor_cmd : Outport
  rudder_cmd : Outport  Port=2
  aileron_cmd : Outport  Port=3
  propeller_cmd : Outport  Port=4
  alt_e : Outport  Port=5
  vel_e : Outport  Port=6
  roll_e : Outport  Port=7
  pitch_e : Outport  Port=8
  wires:
  vel ref/1 -> Velocity Control/1(Velocity Ref)
  altitude ref/1 -> Altitude Control/1(Altitude Ref)
  vel_in/1 -> Velocity Control/2(Velocity)
  Altitude Control/2(altitude_error) -> alt_e/1
  Velocity Control/2(velocity_error) -> vel_e/1
  Altitude Control/1(Pitch_ref) -> Attitude Control/1(Pitch Ref)
  roll_ref/1 -> Attitude Control/2(Roll_ref)
  Euler angles/1 -> Attitude Control/3(Euler angles)
  Attitude Control/1(pitch_error) -> pitch_e/1, Saturation4/1
  Attitude Control/2(roll_error) -> Saturation2/1, roll_e/1
  Velocity Control/1(propeller_cmd) -> Saturation3/1
  Saturation3/1 -> propeller_cmd/1
  Saturation2/1 -> aileron_cmd/1
  Saturation4/1 -> profundor_cmd/1
  altitude/1 -> Altitude Control/2(Altitude)
  Constant/1 -> rudder_cmd/1

== system SIL_OlfatiSaber/UAV 4/Low-level/Guidance Algorithm ==
  yaw : Inport
  x : Inport  Port=2
  y : Inport  Port=3
  x ref : Inport  Port=4
  y ref : Inport  Port=5
  Atan2 : Trigonometry  Operator=atan2
  Constant : Constant
  Constant1 : Constant  Value=0
  Constant2 : Constant  Value=1.2
  Constant3 : Constant  Value=10
  Discrete PID : slpidlib/PID Controller  Controller=PID  Form=Parallel  TimeDomain=Discrete-time  UseExternalTs=off  SampleTime=-1  IntegratorMethod=Forward Euler  FilterMethod=Forward Euler  ControllerParametersSource=external  P=1  I=1  D=0  UseFilter=on  N=100  TunerSelectOption=Transfer Function Based (PID Tuner App)  InitialConditionSource=internal  InitialConditionForIntegrator=0  InitialConditionForFilter=0  DifferentiatorICPrevScaledInput=0  ExternalReset=none  TrackingMode=off  Kt=1  LimitOutput=off  SatLimitsSource=internal  UpperSaturationLimit=inf  LowerSaturationLimit=-inf  LinearizeAsGain=on  AntiWindupMode=none  Kb=1  POutMin=[]  POutMax=[]  IOutMin=[]  IOutMax=[]  DOutMin=[]  DOutMax=[]  NOutMin=[]  NOutMax=[]  SumOutMin=[]  SumOutMax=[]  SaturationOutMin=[]  SaturationOutMax=[]  PParamMin=[]  PParamMax=[]  IParamMin=[]  IParamMax=[]  DParamMin=[]  DParamMax=[]  NParamMin=[]  NParamMax=[]  KbParamMin=[]  KbParamMax=[]  KtParamMin=[]  KtParamMax=[]  KbOutMin=[]  KbOutMax=[]  KtOutMin=[]  KtOutMax=[]  IntegratorOutMin=[]  IntegratorOutMax=[]  FilterOutMin=[]  FilterOutMax=[]  SumI1OutMin=[]  SumI1OutMax=[]  SumI2OutMin=[]  SumI2OutMax=[]  SumI3OutMin=[]  SumI3OutMax=[]  SumI4OutMin=[]  SumI4OutMax=[]  SumDOutMin=[]  SumDOutMax=[]  DifferentiatorOutMin=[]  DifferentiatorOutMax=[]  FilterDiffOutCoefMin=[]  FilterDiffOutCoefMax=[]  ReciprocalOutMin=[]  ReciprocalOutMax=[]  SumDenOutMin=[]  SumDenOutMax=[]  SumNumOutMin=[]  SumNumOutMax=[]  DivideOutMin=[]  DivideOutMax=[]  UdiffTsProdOutMin=[]  UdiffTsProdOutMax=[]  NTsProdOutMin=[]  NTsProdOutMax=[]  UintegralTsProdOutMin=[]  UintegralTsProdOutMax=[]  UngainTsProdOutMin=[]  UngainTsProdOutMax=[]  IntegratorContinuousStateAttributes=''  IntegratorStateMustResolveToSignalObject=off  IntegratorRTWStateStorageClass=Auto  FilterContinuousStateAttributes=''  FilterStateMustResolveToSignalObject=off  FilterRTWStateStorageClass=Auto  ParallelPVariant=ExternalParameters  IdealPVariant=Disabled  IVariant=ExternalParameters  DVariant=ExternalParameters  IntegratorVariant=Discrete  SatVariant=Disabled  AWVariant=Passthrough  PCopyVariant=Disabled  TRVariant=Disabled  FdbkBlocksVariant=Forward  IdealPFdbkVariant=Disabled  SatFdbkVariant=Disabled  DerivativeFilterVariant=ForwardEulerFilter  NVariant=ExternalParameters  NCopyVariant=Disabled  FilterICVariant=InternalICsFilter  IntegratorICVariant=InternalICs  ExternalResetVariant=Disabled  TRSumVariant=Passthrough  SumFdbkVariant=Disabled  SumVariant=Sum_PID  TsampFilterVariant=InternalTs  TsampNgainVariant=Passthrough  TsampIntegralVariant=Passthrough  ExternalSaturationOutDataTypeStr=Inherit: Same as second input
  Gain : Gain  Gain=1.67
  Gain1 : Gain  Gain=-1
  Mux1 : Mux  Inputs=2
  Mux2 : Mux  Inputs=2
  Mux3 : Mux  Inputs=2
  Saturation : Saturate  UpperLimit=0.226893  LowerLimit=-0.226893
  Sum2 : Sum  Inputs=|+-
  Sum3 : Sum  Inputs=|+-
  Sum4 : Sum  Inputs=|+-
  roll_ref : Outport
  yaw_error : Outport  Port=2
  positions : Outport  Port=3
  wires:
  Mux1/1 -> Mux3/1
  Mux2/1 -> Mux3/2
  Saturation/1 -> Gain1/1
  Sum3/1 -> Atan2/1
  y/1 -> Sum3/2, Mux2/2
  y ref/1 -> Mux2/1, Sum3/1
  x ref/1 -> Mux1/1, Sum2/1
  x/1 -> Sum2/2, Mux1/2
  Sum2/1 -> Atan2/2
  Atan2/1 -> Sum4/1
  yaw/1 -> Sum4/2
  Mux3/1 -> positions/1
  Discrete PID/1 -> Saturation/1
  Sum4/1 -> yaw_error/1, Gain/1
  Gain1/1 -> roll_ref/1
  Constant/1 -> Discrete PID/2
  Constant1/1 -> Discrete PID/3
  Constant2/1 -> Discrete PID/4
  Constant3/1 -> Discrete PID/5
  Gain/1 -> Discrete PID/1

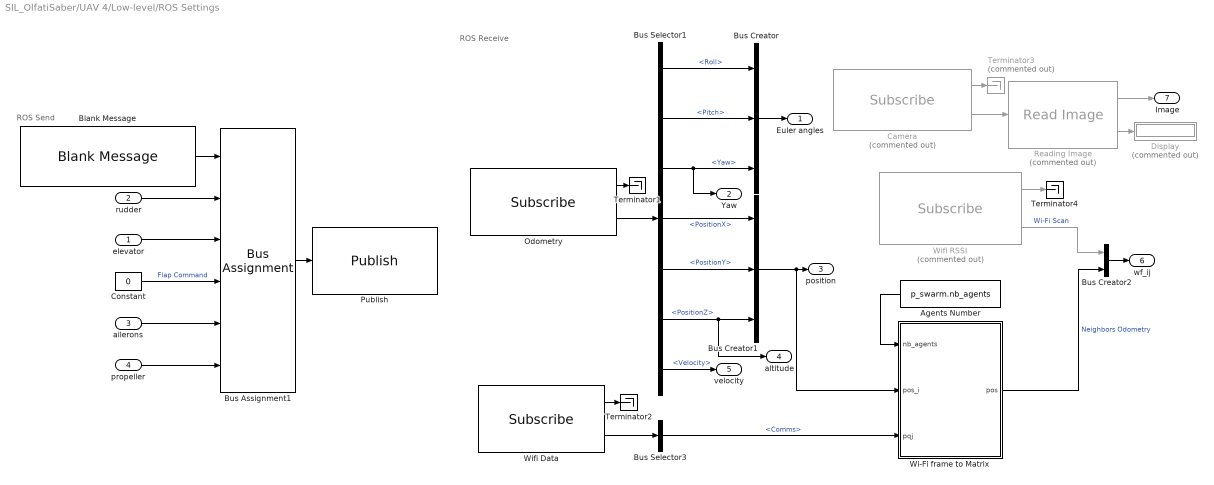
== system SIL_OlfatiSaber/UAV 4/Low-level/ROS Settings ==
  note: ROS Receive
  note: ROS Send
  elevator : Inport
  rudder : Inport  Port=2
  ailerons : Inport  Port=3
  propeller : Inport  Port=4
  Agents Number : Constant  Value=p_swarm.nb_agents
  Blank Message : robotlib/Blank Message  messageClass=Message  entityType=cosmus_messages/Control_Surfaces  messageType=cosmus_messages/Control_Surfaces  SampleTime=-1  legacyBusStruct=off
  Bus Assignment1 : BusAssignment  AssignedSignals=Rudder,Elevators,RightFlap,RightAileron,Propeller
  Bus Creator : BusCreator  Inputs=3
  Bus Creator1 : BusCreator  Inputs=3
  Bus Creator2 : BusCreator  Inputs=2
  Bus Selector1 : BusSelector  OutputSignals=Roll,Pitch,Yaw,PositionX,PositionY,PositionZ,Velocity
  Bus Selector3 : BusSelector  OutputSignals=Comms
  Camera : robotlib/Subscribe  Commented=on  topicSource=Select from ROS network  topic=/uav1/camera/image_raw  messageType=sensor_msgs/Image  SampleTime=-1  legacyBusStruct=off  messageQueueLength=1
  Constant : Constant  Value=0
  Display : Display  Commented=on
  Odometry : robotlib/Subscribe  topicSource=Select from ROS network  topic=/uav4/ground_truth/Odometry  messageType=cosmus_communication/Odom  SampleTime=-1  legacyBusStruct=off  messageQueueLength=1
  Publish : robotlib/Publish  topicSource=Select from ROS network  topic=/uav4/command  messageType=cosmus_messages/Control_Surfaces  legacyBusStruct=off  messageQueueLength=1
  Reading Image : robotlib/Read Image  Commented=on  MaximumImageSize=[240, 360]  ImageEncoding=rgb8  ShowAlphaOutput=off  ShowErrorCodeOutput=on  VariableSizeOutputs=off
      settings: SourceProductBaseCode=RR
  Terminator1 : Terminator
  Terminator2 : Terminator
  Terminator3 : Terminator  Commented=on
  Terminator4 : Terminator
  Wi-Fi frame to Matrix : MATLAB Function  TreatAsAtomicUnit=on
  Wifi Data : robotlib/Subscribe  topicSource=Select from ROS network  topic=/uav4/wifi_receiver/data  messageType=cosmus_messages/NetworkComm  SampleTime=-1  legacyBusStruct=off  messageQueueLength=1
  Wifi RSSI : robotlib/Subscribe  Commented=on  topicSource=Select from ROS network  topic=/uav1/wifi_receiver/wifi_scan  messageType=cosmus_messages/WifiSignals  SampleTime=-1  legacyBusStruct=off  messageQueueLength=1
  Euler angles : Outport
  Yaw : Outport  Port=2
  position : Outport  Port=3
  altitude : Outport  Port=4
  velocity : Outport  Port=5
  wf_ij : Outport  Port=6
  Image : Outport  Port=7
  wires:
  Odometry/1 -> Terminator1/1
  Blank Message/1 -> Bus Assignment1/1
  Bus Selector1/3 -> Bus Creator/3, Yaw/1  "<Yaw>"
  Bus Creator/1 -> Euler angles/1
  Bus Selector1/1 -> Bus Creator/1  "<Roll>"
  Bus Selector1/2 -> Bus Creator/2  "<Pitch>"
  Constant/1 -> Bus Assignment1/4  "Flap Command"
  Bus Assignment1/1 -> Publish/1
  Odometry/2 -> Bus Selector1/1
  Bus Selector1/4 -> Bus Creator1/1  "<PositionX>"
  Bus Selector1/5 -> Bus Creator1/2  "<PositionY>"
  Bus Selector1/6 -> Bus Creator1/3, altitude/1  "<PositionZ>"
  propeller/1 -> Bus Assignment1/6
  ailerons/1 -> Bus Assignment1/5
  elevator/1 -> Bus Assignment1/3
  Bus Selector1/7 -> velocity/1  "<Velocity>"
  rudder/1 -> Bus Assignment1/2
  Wifi Data/1 -> Terminator2/1
  Wifi Data/2 -> Bus Selector3/1
  Bus Selector3/1 -> Wi-Fi frame to Matrix/3(pqj)  "<Comms>"
  Agents Number/1 -> Wi-Fi frame to Matrix/1(nb_agents)
  Bus Creator1/1 -> position/1, Wi-Fi frame to Matrix/2(pos_i)
  Wi-Fi frame to Matrix/1(pos) -> Bus Creator2/2  "Neighbors Odometry"
  Camera/2 -> Reading Image/1
  Reading Image/1 -> Image/1
  Reading Image/2 -> Display/1
  Camera/1 -> Terminator3/1
  Wifi RSSI/1 -> Terminator4/1
  Wifi RSSI/2 -> Bus Creator2/1  "Wi-Fi Scan"
  Bus Creator2/1 -> wf_ij/1

== system SIL_OlfatiSaber/UAV 4/Low-level/Vision ==
  Image : Inport
  Video Viewer : VideoViewer  Commented=on  FigPos=[505 744 418 304]
  wires:
  Image/1 -> Video Viewer/1

== system SIL_OlfatiSaber/UAV 5/High-level/Coordination Algorithm ==
  Xi : Inport
  u : Inport  Port=2
  Demux : Demux  Outputs=3
  Discrete Derivative : simulink/Discrete/Discrete Derivative  gainval=1.0  ICPrevScaledInput=0.0  OutMin=[]  OutMax=[]  OutDataType=fixdt(1, 16)  OutScaling=2^-10  DoSatur=off
  Discrete-Time Integrator : DiscreteIntegrator  SampleTime=-1  ICPrevOutput=DiscIntNeverNeededParam  ICPrevScaledInput=DiscIntNeverNeededParam
  Olfati-Saber Algorithm : MATLAB Function  TreatAsAtomicUnit=on
  Parameters : Subsystem
  dt : Constant  Value=0.01
  r_agent : Constant  Value=p_swarm.r_agent
  X : Outport
  Y : Outport  Port=2
  Z : Outport  Port=3
  wires:
  Olfati-Saber Algorithm/1(vel_command) -> Discrete-Time Integrator/1
  dt/1 -> Olfati-Saber Algorithm/5(dt)
  r_agent/1 -> Olfati-Saber Algorithm/6(r_agent)
  Discrete-Time Integrator/1 -> Demux/1
  Demux/2 -> Y/1
  Demux/1 -> X/1
  Demux/3 -> Z/1
  Discrete Derivative/1 -> Olfati-Saber Algorithm/3(vel)
  Parameters/1(p_swarm) -> Olfati-Saber Algorithm/1(p_swarm_par)
  Xi/1 -> Discrete Derivative/1, Olfati-Saber Algorithm/2(pos)
  u/1 -> Olfati-Saber Algorithm/4(u_ref)

== system SIL_OlfatiSaber/UAV 5/High-level/Network ==
  Scan : Inport
  Agents Number : Constant  Value=p_swarm.nb_agents
  Bus Selector : BusSelector  OutputSignals=Neighbors Odometry,Wi-Fi Scan
  Status Network : MATLAB Function  Commented=on  TreatAsAtomicUnit=on
  Terminator5 : Terminator
  Pos_J : Outport
  wires:
  Status Network/1(SignalDbms) -> Terminator5/1
  Agents Number/1 -> Status Network/1(N_Agents)
  Scan/1 -> Bus Selector/1
  Bus Selector/1 -> Pos_J/1  "<Neighbors Odometry>"
  Bus Selector/2 -> Status Network/2(Wifi_Scan)  "<Wi-Fi Scan>"

== system SIL_OlfatiSaber/UAV 5/High-level/Waypoint Generator ==
  Xi : Inport
  Pos_i : Inport  Port=2
  Constant : Constant  Value=radius_waypoint
  Constant1 : Constant  Value=Waypoints
  Constant2 : Constant  Value=N_Waypoints
  Constant3 : Constant  Value=p_swarm.r
  Display : Display
  Memory : Memory
  Velocity Direction : MATLAB Function  TreatAsAtomicUnit=on
  Waypoint Algorithm : MATLAB Function  TreatAsAtomicUnit=on
  u : Outport
  wires:
  Memory/1 -> Waypoint Algorithm/6("Current_Waypoint ")
  Constant1/1 -> Waypoint Algorithm/4(Waypoints)
  Xi/1 -> Waypoint Algorithm/1(Xi)
  Constant3/1 -> Waypoint Algorithm/3(p_swarm_r)
  Constant2/1 -> Waypoint Algorithm/5(N_Waypoints)
  Waypoint Algorithm/2(Current_Waypoint) -> Memory/1, Display/1
  Constant/1 -> Waypoint Algorithm/2(R)
  Pos_i/1 -> Velocity Direction/1(pos)
  Velocity Direction/1(u_ref) -> u/1
  Waypoint Algorithm/1(wp) -> Velocity Direction/2(wp)

== system SIL_OlfatiSaber/UAV 5/Low-level/Autopilot ==
  note: bota po
  vel ref : Inport
  Euler angles : Inport  Port=2
  roll_ref : Inport  Port=3
  altitude : Inport  Port=4
  vel_in : Inport  Port=5
  altitude ref : Inport  Port=6
  Altitude Control : Subsystem
      settings: PortSchema="{\"entries\":[{\"content\":{\"sides\":[{\"content\":{\"connectorIds\":[\"In1\",\"In2\"]},\"type\":\"ConnectorPlacement.EquallySpacedRectSide\",\"uuid\":\"98c80c82-2588-492a-897d-d133440579b3\"},{\"content\":{\"connectorIds\":[\"Out1\"],\"side\":\"RIGHT\"},\"type\":\"ConnectorPlacement.EquallySpacedRectSide\",\"uuid\":\"157fcffb-564d-4941-a636-42e4165df758\"},{\"content\":{\"connectorIds\":[\"Out2\"],\"side\":\"TOP\"},\"type\":\"ConnectorPlacement.EquallySpacedRectSide\",\"uuid\":\"44b57248-226e-45fd-814c-d7eb072c2d1f\"},{\"content\":{\"connectorIds\":[],\"side\":\"HIDDEN\"},\"type\":\"ConnectorPlacement.EquallySpacedRectSide\",\"uuid\":\"dff6d6ab-ae11-4516-9107-00b7ae45fb5b\"}]},\"type\":\"ConnectorPlacement.EquallySpacedConnector\",\"uuid\":\"b6a62117-e3d4-4c2a-a3b5-b134a2ba950a\"}],\"packageUris\":[\"http://schema.mathworks.com/mf0/Connector/R2020b\"],\"version\":\"1.0\"}"
  Attitude Control : Subsystem
  Constant : Constant  Value=0
  Saturation2 : Saturate  UpperLimit=0.0523599  LowerLimit=-0.0523599
  Saturation3 : Saturate  UpperLimit=0.8  LowerLimit=0.6
  Saturation4 : Saturate  UpperLimit=0.0523599  LowerLimit=-0.0523599
  Takeoff : Subsystem  Commented=on
  Velocity Control : Subsystem
      settings: PortSchema="{\"entries\":[{\"content\":{\"sides\":[{\"content\":{\"connectorIds\":[\"In1\",\"In2\"]},\"type\":\"ConnectorPlacement.EquallySpacedRectSide\",\"uuid\":\"98c80c82-2588-492a-897d-d133440579b3\"},{\"content\":{\"connectorIds\":[\"Out1\"],\"side\":\"RIGHT\"},\"type\":\"ConnectorPlacement.EquallySpacedRectSide\",\"uuid\":\"157fcffb-564d-4941-a636-42e4165df758\"},{\"content\":{\"connectorIds\":[\"Out2\"],\"side\":\"TOP\"},\"type\":\"ConnectorPlacement.EquallySpacedRectSide\",\"uuid\":\"44b57248-226e-45fd-814c-d7eb072c2d1f\"},{\"content\":{\"connectorIds\":[],\"side\":\"HIDDEN\"},\"type\":\"ConnectorPlacement.EquallySpacedRectSide\",\"uuid\":\"dff6d6ab-ae11-4516-9107-00b7ae45fb5b\"}]},\"type\":\"ConnectorPlacement.EquallySpacedConnector\",\"uuid\":\"b6a62117-e3d4-4c2a-a3b5-b134a2ba950a\"}],\"packageUris\":[\"http://schema.mathworks.com/mf0/Connector/R2020b\"],\"version\":\"1.0\"}"
  profundor_cmd : Outport
  rudder_cmd : Outport  Port=2
  aileron_cmd : Outport  Port=3
  propeller_cmd : Outport  Port=4
  alt_e : Outport  Port=5
  vel_e : Outport  Port=6
  roll_e : Outport  Port=7
  pitch_e : Outport  Port=8
  wires:
  vel ref/1 -> Velocity Control/1(Velocity Ref)
  altitude ref/1 -> Altitude Control/1(Altitude Ref)
  vel_in/1 -> Velocity Control/2(Velocity)
  Altitude Control/2(altitude_error) -> alt_e/1
  Velocity Control/2(velocity_error) -> vel_e/1
  Altitude Control/1(Pitch_ref) -> Attitude Control/1(Pitch Ref)
  roll_ref/1 -> Attitude Control/2(Roll_ref)
  Euler angles/1 -> Attitude Control/3(Euler angles)
  Attitude Control/1(pitch_error) -> pitch_e/1, Saturation4/1
  Attitude Control/2(roll_error) -> Saturation2/1, roll_e/1
  Velocity Control/1(propeller_cmd) -> Saturation3/1
  Saturation3/1 -> propeller_cmd/1
  Saturation2/1 -> aileron_cmd/1
  Saturation4/1 -> profundor_cmd/1
  altitude/1 -> Altitude Control/2(Altitude)
  Constant/1 -> rudder_cmd/1
